simulink model "NonlinearModel"  (R2022b)
settings: Solver=VariableStepAuto  StartTime=0.0  StopTime=10.0  RelTol=1e-3
undefined symbols (not defined in the file): C_pid, Cz_euler, Cz_zoh, init, theta_l_init, vision_fps
libraries: simulink x1
settings Model: Creator=tumisangramotlhwa  LastModifiedBy=tumisangramotlhwa

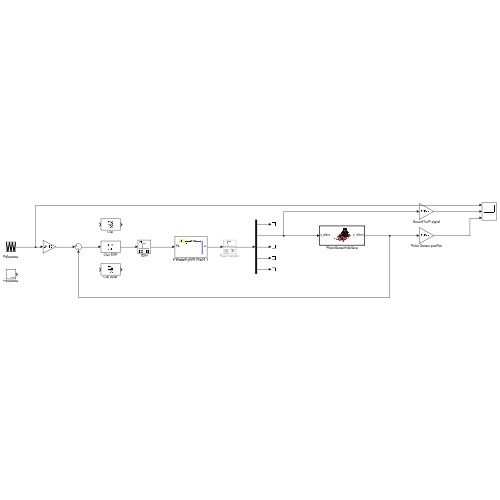
[thumbnail: Simulink's stored preview of the top-level diagram]
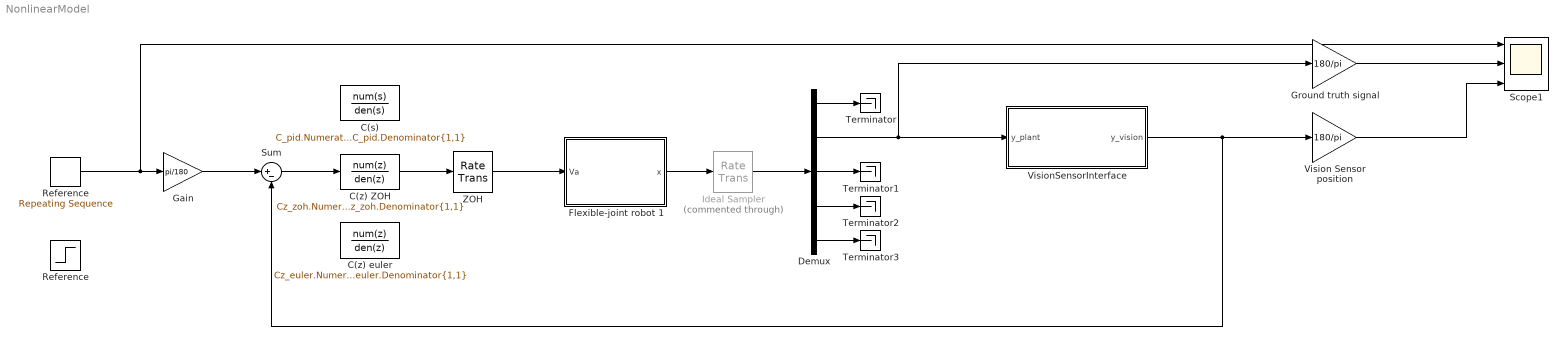
== system NonlinearModel ==
  " Reference" : simulink/Sources/Repeating Sequence  rep_seq_t=[0 2 4]  rep_seq_y=[45 15 45]
  C(s) : TransferFcn  Numerator=C_pid.Numerator{1,1}  Denominator=C_pid.Denominator{1,1}
  C(z) ZOH : DiscreteTransferFcn  Numerator=Cz_zoh.Numerator{1,1}  Denominator=Cz_zoh.Denominator{1,1}
  C(z) euler : DiscreteTransferFcn  Numerator=Cz_euler.Numerator{1,1}  Denominator=Cz_euler.Denominator{1,1}
  Demux : Demux  Outputs=5
  Flexible-joint robot 1 : Subsystem
      mask Display: image('$imagefile'); % Use "Edit Image" on toolstrip to change.
  Gain : Gain  Gain=pi/180
  Ground truth signal : Gain  Gain=180/pi
  Ideal Sampler : RateTransition  Commented=through  OutPortSampleTime=Ts
  Reference : Step  Time=5  Before=45  After=15  SampleTime=0
  Scope1 : Scope  NumInputPorts=3
  Sum : Sum  Inputs=|+-
  Terminator{,1..3} (4 alike) : Terminator
  Vision Sensor position : Gain  Gain=180/pi
  VisionSensorInterface : Subsystem  TreatAsAtomicUnit=on
      mask Display: image('$imagefile'); % Use "Edit Image" on toolstrip to change.
  ZOH : RateTransition
  wires:
  " Reference"/1 -> Scope1/1, Gain/1
  Gain/1 -> Sum/1
  ZOH/1 -> Flexible-joint robot 1/1(Va)
  Sum/1 -> C(z) ZOH/1
  C(z) ZOH/1 -> ZOH/1
  Demux/2 -> Ground truth signal/1, VisionSensorInterface/1(y_plant)
  Demux/5 -> Terminator3/1
  Demux/4 -> Terminator2/1
  Demux/3 -> Terminator1/1
  Demux/1 -> Terminator/1
  VisionSensorInterface/1(y_vision) -> Vision Sensor position/1, Sum/2
  Flexible-joint robot 1/1(x) -> Ideal Sampler/1
  Ground truth signal/1 -> Scope1/2
  Vision Sensor position/1 -> Scope1/3
  Ideal Sampler/1 -> Demux/1

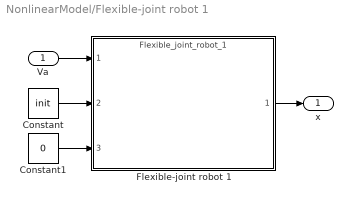
== system NonlinearModel/Flexible-joint robot 1 ==
  Va : Inport
  Constant : Constant  Value=init
  Constant1 : Constant  Value=0
  Flexible-joint robot 1 : ModelReference  ModelNameDialog=Flexible_joint_robot_1  ModelReferenceVersion=1.63  CopyOfModelProtected=on
  x : Outport
  wires:
  Constant/1 -> Flexible-joint robot 1/2
  Constant1/1 -> Flexible-joint robot 1/3
  Flexible-joint robot 1/1 -> x/1
  Va/1 -> Flexible-joint robot 1/1

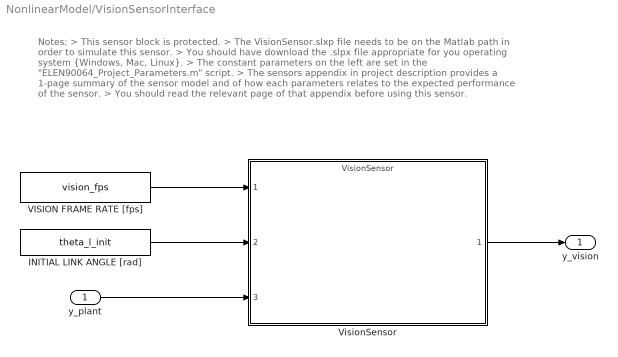
== system NonlinearModel/VisionSensorInterface ==
  note: Notes:
      | > This sensor block is protected.
      | > The VisionSensor.slxp file needs to be on the Matlab path in order to simulate this sensor.
      | > You should have download the .slpx file appropriate for you operating system {Windows, Mac, Linux}.
      | > The constant parameters on the left are set in the "ELEN90064_Project_Parameters.m" script.
      | > The sensors appendix in project description provides a 1-page summary of the sensor model and of how each parameters relates to the expected performance of the sensor.
      | > You should read the relevant page of that appendix before using this sensor.
  y_plant : Inport
  INITIAL LINK ANGLE [rad] : Constant  Value=theta_l_init
  VISION FRAME RATE [fps] : Constant  Value=vision_fps
  VisionSensor : ModelReference  ModelNameDialog=VisionSensor.slxp  ModelReferenceVersion=1.19  CopyOfModelProtected=on
  y_vision : Outport
  wires:
  VISION FRAME RATE [fps]/1 -> VisionSensor/1
  INITIAL LINK ANGLE [rad]/1 -> VisionSensor/2
  y_plant/1 -> VisionSensor/3
  VisionSensor/1 -> y_vision/1
